simulink model "PlateauSim_Opti"  (R2019b)
settings: Solver=FixedStepAuto  StartTime=0.0  StopTime=165  RelTol=1e-3
values from neighbouring files (symbols this model uses):
  Abs2Dna = ConversionFactor*Reactor_Volume    (= 1250)    [ParameterEstimation.m]    (also in PlateauSimCode.m; ReactorModel_code.m)
  Dna2Abs = 1/Abs2Dna    (= 0.0008)    [ParameterEstimation.m]    (also in PlateauSimCode.m; ReactorModel_code.m)
  kd = Fitdat{8,col}{strcmp(Fitdat{8,col}.Param, 'k'), 2}    [Excel_Import.m]    (also in Matlab_YM_anno.m = DNaseParam{strcmp(DNaseParam.Param, 'k'), 2}; ParameterEstimation.m = 0.05; PlateauSimCode.m = EstParam{cfit,'kd'}{1,1}; ReactorModel_code.m = EstParam{cfit,'kd'})
  kn = Fitdat{6,col}{strcmp(Fitdat{6,col}.Param, 'k'), 2}    [Excel_Import.m]    (also in Matlab_YM_anno.m = NaDeoParam{strcmp(NaDeoParam.Param, 'k'), 2}; ParameterEstimation.m = 0.05; PlateauSimCode.m = EstParam{cfit,'kn'}{1,1}; ReactorModel_code.m = EstParam{cfit,'kn'}{1,1})
  MaxD = 0.5    [ParameterEstimation.m]    (also in PlateauSimCode.m = EstParam{cfit,'MaxD'}{1,1}; ReactorModel_code.m = EstParam{cfit,'MaxD'})
  MaxN = 0.5    [ParameterEstimation.m]    (also in PlateauSimCode.m = EstParam{cfit,'MaxN'}{1,1}; ReactorModel_code.m = EstParam{cfit,'MaxN'})
  td0 = tnend+twash    [ParameterEstimation.m]    (also in PlateauSimCode.m; ReactorModel_code.m)
  tn0 = 0    [ParameterEstimation.m]    (also in PlateauSimCode.m; ReactorModel_code.m)
  TotalDNA = 100    [FIgure_Test.m]    (also in ParameterEstimation.m = DNA*Mass_ECM_dry; PlateauSimCode.m = DNA*Mass_ECM_dry; ReactorModel_code.m = DNA*Mass_ECM_dry)
  y0d = 0    [Excel_Import.m]    (also in Matlab_YM_anno.m; ParameterEstimation.m; PlateauSimCode.m; ReactorModel_code.m)
  y0n = 0    [Excel_Import.m]    (also in Matlab_YM_anno.m; ParameterEstimation.m; PlateauSimCode.m; ReactorModel_code.m)
libraries: simulink x2
settings Model: OrderedModelArguments=off  Creator=daphnesze  LastModifiedBy=daphnesze
settings DataIOCC: OutputOption=AdditionalOutputTimes  OutputTimes=SDO_OutputTimes  ReturnWorkspaceOutputsName=SDOSimTest_Log
settings OptimizationCC: BlockReduction=off  DefaultParameterBehavior=Inlined  BufferReuse=off

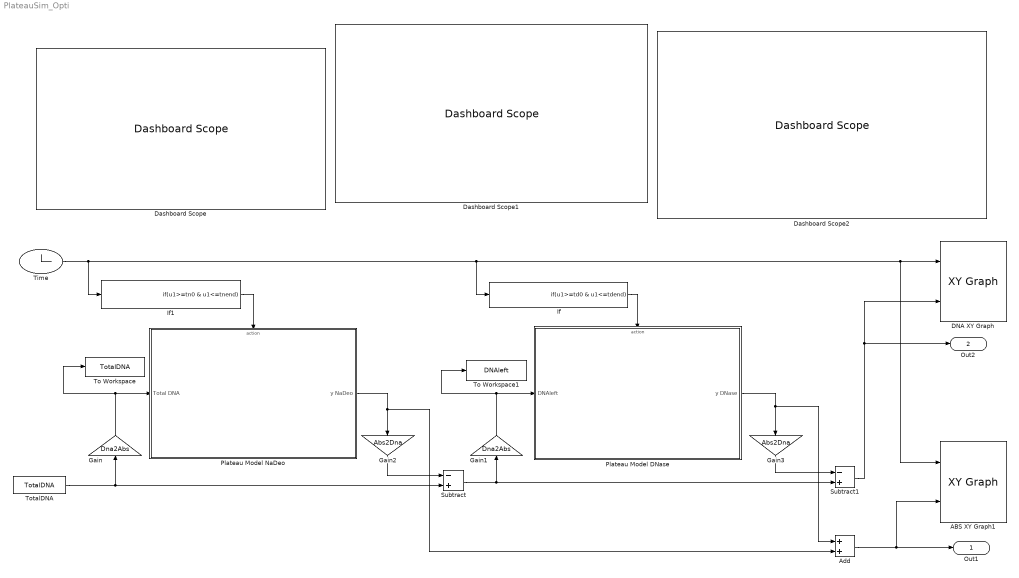
== system PlateauSim_Opti ==
  ABS XY Graph1 : simulink/Sinks/XY Graph  xmin=0  xmax=tdend  ymin=0  ymax=5  st=-1
  Add : Sum
  DNA XY Graph : simulink/Sinks/XY Graph  xmin=0  xmax=tdend  ymin=0  ymax=TotalDNA  st=-1
  Dashboard Scope : DashboardScope
  Dashboard Scope1 : DashboardScope
  Dashboard Scope2 : DashboardScope
  Gain : Gain  Gain=Dna2Abs
  Gain1 : Gain  Gain=Dna2Abs
  Gain2 : Gain  Gain=Abs2Dna
  Gain3 : Gain  Gain=Abs2Dna
  If : If  IfExpression=u1>=td0 & u1<=tdend  ShowElse=off
  If1 : If  IfExpression=u1>=tn0 & u1<=tnend  ShowElse=off
  "Plateau Model DNase " : Subsystem  TreatAsAtomicUnit=on
  Plateau Model NaDeo : Subsystem  TreatAsAtomicUnit=on
  Subtract : Sum  Inputs=-+
  Subtract1 : Sum  Inputs=-+
  Time : Clock
  To Workspace : ToWorkspace  VariableName=TotalDNA  SampleTime=-1
  To Workspace1 : ToWorkspace  VariableName=DNAleft  SampleTime=-1
  TotalDNA : Constant  Value=TotalDNA
  Out1 : Outport  SignalName=Abs
  Out2 : Outport  Port=2  SignalName=DNA
  wires:
  Time/1 -> If1/1, If/1, ABS XY Graph1/1, DNA XY Graph/1
  If1/1 -> Plateau Model NaDeo/Action
  TotalDNA/1 -> Subtract/2, Gain/1
  Plateau Model NaDeo/1("y NaDeo ") -> Add/2, Gain2/1
  If/1 -> "Plateau Model DNase "/Action
  "Plateau Model DNase "/1("y DNase ") -> Add/1, Gain3/1
  Subtract1/1 -> DNA XY Graph/2, Out2/1
  Gain/1 -> To Workspace/1, Plateau Model NaDeo/1(Total DNA)
  Gain1/1 -> To Workspace1/1, "Plateau Model DNase "/1(DNAleft)
  Gain2/1 -> Subtract/1
  Gain3/1 -> Subtract1/1
  Add/1 -> ABS XY Graph1/2, Out1/1
  Subtract/1 -> Subtract1/2, Gain1/1

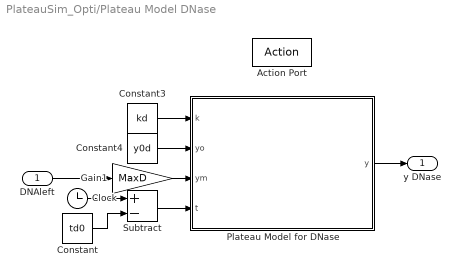
== system PlateauSim_Opti/Plateau Model DNase  ==
  DNAleft : Inport
  Action Port : ActionPort  InitializeStates=reset  PropagateVarSize=During execution  ActionPortLabel=if(u1>=td0 & u1<=tdend)
  Clock : Clock
  Constant : Constant  Value=td0
  Constant3 : Constant  Value=kd
  Constant4 : Constant  Value=y0d
  Gain1 : Gain  Gain=MaxD  ParamMin=0  ParamMax=1
  Plateau Model for DNase : MATLAB Function  TreatAsAtomicUnit=on
  Subtract : Sum  Inputs=+-
  "y DNase " : Outport
  wires:
  Gain1/1 -> Plateau Model for DNase/3(ym)
  Constant3/1 -> Plateau Model for DNase/1(k)
  Constant4/1 -> Plateau Model for DNase/2(yo)
  DNAleft/1 -> Gain1/1
  Clock/1 -> Subtract/1
  Subtract/1 -> Plateau Model for DNase/4(t)
  Plateau Model for DNase/1(y) -> "y DNase "/1
  Constant/1 -> Subtract/2

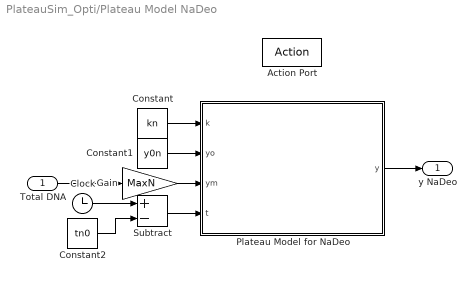
== system PlateauSim_Opti/Plateau Model NaDeo ==
  Total DNA : Inport
  Action Port : ActionPort  InitializeStates=reset  PropagateVarSize=During execution  ActionPortLabel=if(u1>=tn0 & u1<=tnend)
  Clock : Clock
  Constant : Constant  Value=kn
  Constant1 : Constant  Value=y0n
  Constant2 : Constant  Value=tn0
  Gain : Gain  Gain=MaxN  ParamMin=0  ParamMax=1
  Plateau Model for NaDeo : MATLAB Function  TreatAsAtomicUnit=on
  Subtract : Sum  Inputs=+-
  "y NaDeo " : Outport
  wires:
  Gain/1 -> Plateau Model for NaDeo/3(ym)
  Constant1/1 -> Plateau Model for NaDeo/2(yo)
  Constant/1 -> Plateau Model for NaDeo/1(k)
  Total DNA/1 -> Gain/1
  Subtract/1 -> Plateau Model for NaDeo/4(t)
  Plateau Model for NaDeo/1(y) -> "y NaDeo "/1
  Constant2/1 -> Subtract/2
  Clock/1 -> Subtract/1

== matlab function PlateauSim_Opti/Plateau Model DNase /Plateau Model for DNase ==
  data: k input; y output; yo input; ym input; t input

function y  = BioReactor_model(k,yo,ym,t)
[y] = ym-(ym-yo)*exp((-k)*t);
end

== matlab function PlateauSim_Opti/Plateau Model NaDeo/Plateau Model for NaDeo ==
  data: k input; y output; yo input; ym input; t input

function y  = BioReactor_model(k,yo,ym,t)
[y] = ym-(ym-yo)*exp((-k)*t);
end
